simulink model "xpc1_rlti_varx_sqrt"  (Simulink 7.8)
settings: Solver=FixedStepDiscrete  StartTime=0.0  StopTime=150.0  FixedStep=0.005  RelTol=1e-3
libraries: xpclib x3, cstblocks x2, xpcnilib x2, simulink x1
settings Model: Creator=IVO  LastModifiedBy=pietergebraad  SimulationMode=external  BufferReuse=off
settings OptimizationCC: BlockReduction=off  OptimizeBlockIOStorage=off  BufferReuse=off  ExpressionFolding=off  LocalBlockOutputs=off
settings DebuggingCC: FcnCallInpInsideContextMsg=Use local settings  StrictBusMsg=Warning
settings HardwareCC: ProdIntDivRoundTo=Zero  ProdEndianess=LittleEndian  ProdHWDeviceType=Generic->32-bit x86 compatible
settings SFSimCC: SFSimEnableDebug=off  SimParseCustomCode=off
settings RTWCC: SystemTargetFile=xpctarget.tlc  TemplateMakefile=xpc_default_tmf  Description=xPC Target  ProcessScript=xpctarget_make_rtw_hook  RTWCompilerOptimization=On
settings xpcTargetCC: TargetFcnLib=ansi_tfl_table_tmw.mat  TargetFunctionLibrary=XPC_BLAS  CodeExecutionProfiling=off  ParMdlRefBuildCompliant=on  ConcurrentExecutionCompliant=on  CombineSignalStateStructs=off  PortableWordSizes=off  xPCTaskExecutionProfile=off  xPCRL32EventNumber=5000  xPCisDefaultEnv=off  xPCTargetPCEnvName=TargetPC1  xPCLoadParamSetFile=off  xPCConcurrentTasks=off  xPCEnableSFAnimation=off

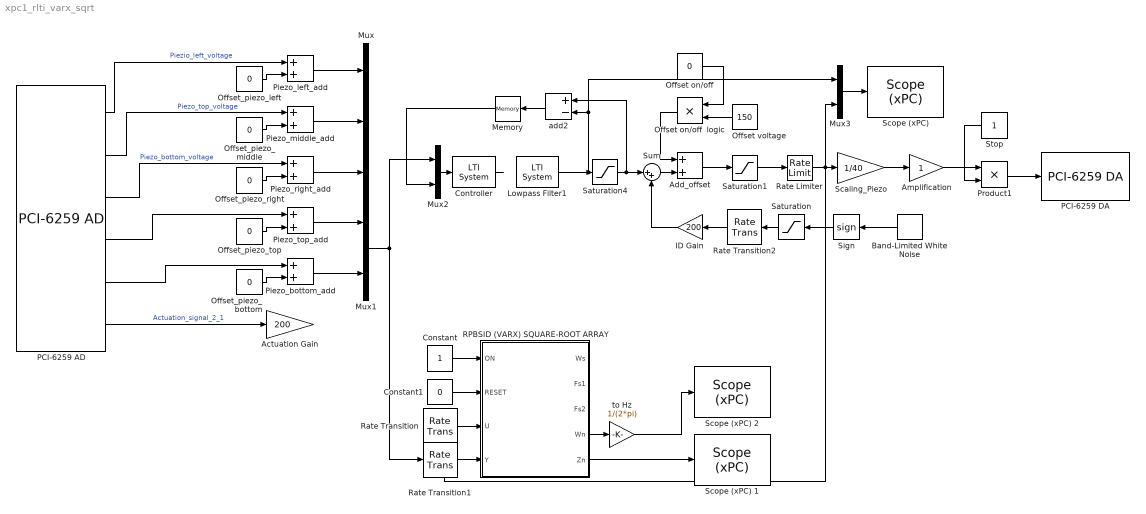
== system xpc1_rlti_varx_sqrt ==
  Actuation Gain : Gain  Gain=200
  Add_offset : Sum
  Amplification : Gain
  Band-Limited White Noise : simulink/Sources/Band-Limited White Noise  Cov=1  Ts=0.25  seed=[23341]
  Constant : Constant
  Constant1 : Constant  Value=0
  Controller : cstblocks/LTI System  sys=Cs  IC=[]
  ID Gain : Gain  Gain=200
  Lowpass Filter1 : cstblocks/LTI System  sys=Fs  IC=[]
  Memory : Memory
  Mux : Mux  Inputs=3
  Mux1 : Mux  Inputs=2
  Mux2 : Mux  Inputs=2
  Mux3 : Mux  Inputs=2
  Offset on/off : Constant  Value=0  OutDataTypeStr=boolean
  Offset on/off  logic : Product  RndMeth=Zero
  Offset voltage : Constant  Value=150
  Offset_piezo_bottom : Constant  Value=0
  Offset_piezo_left : Constant  Value=0
  Offset_piezo_middle : Constant  Value=0
  Offset_piezo_right : Constant  Value=0
  Offset_piezo_top : Constant  Value=0
  PCI-6259 AD : xpcnilib/A//D/M Series/PCI-6259 AD  channel=[17,18,19,20,21,22]  range=[10]  coupling=[0]  scantime=5e-6  sampletime=0.005  slot=-1
  PCI-6259 DA : xpcnilib/D//A/M Series/PCI-6259 DA  channel=[3]  range=[10]  reset=[1]  initValue=[0]  sampletime=0.005  slot=-1
  Piezo_bottom_add : Sum
  Piezo_left_add : Sum
  Piezo_middle_add : Sum
  Piezo_right_add : Sum
  Piezo_top_add : Sum
  Product1 : Product  RndMeth=Zero
  RPBSID (VARX) SQUARE-ROOT ARRAY : MATLAB Function  TreatAsAtomicUnit=on
  Rate Limiter : RateLimiter  RisingSlewLimit=10000  FallingSlewLimit=-10000  SampleTimeMode=inherited
  Rate Transition : RateTransition  Integrity=off  Deterministic=off  OutPortSampleTime=0.05
  Rate Transition1 : RateTransition  Integrity=off  Deterministic=off  OutPortSampleTime=0.05
  Rate Transition2 : RateTransition
  Saturation : Saturate  UpperLimit=1  LowerLimit=-1
  Saturation1 : Saturate  UpperLimit=290  LowerLimit=-290
  Saturation4 : Saturate  UpperLimit=290  LowerLimit=-290
  Scaling_Piezo : Gain  Gain=1/40
  "Scope (xPC) " : xpclib/Misc./Scope (xPC)   scopeno=1  scopetype=Target  autostart=on  viewmode=Graphical rolling  formatstr='%15.6f'  grid=on  ylimits=[-300,300]  nosamples=600  noprepostsamples=0  interleave=1  triggermode=FreeRun  triggersignal=1  triggerlevel=0.0  triggerslope=Either  triggerscope=1  triggersample=0  filename=data.dat  mode=Lazy  writesize=512  autorestart=off  dynamicfilemode=off  maxwritefilesize=512*1024^2
  Scope (xPC) 1 : xpclib/Misc./Scope (xPC)   scopeno=2  scopetype=Target  autostart=on  viewmode=Graphical rolling  formatstr='%15.6f'  grid=on  ylimits=[-0.05,0.03]  nosamples=60  noprepostsamples=0  interleave=1  triggermode=FreeRun  triggersignal=1  triggerlevel=0.0  triggerslope=Either  triggerscope=1  triggersample=0  filename=data.dat  mode=Lazy  writesize=512  autorestart=off  dynamicfilemode=off  maxwritefilesize=512*1024^2
  Scope (xPC) 2 : xpclib/Misc./Scope (xPC)   scopeno=3  scopetype=Target  autostart=on  viewmode=Graphical rolling  formatstr='%15.6f'  grid=on  ylimits=[2,3.5]  nosamples=60  noprepostsamples=0  interleave=1  triggermode=FreeRun  triggersignal=1  triggerlevel=0.0  triggerslope=Either  triggerscope=1  triggersample=0  filename=data.dat  mode=Lazy  writesize=512  autorestart=off  dynamicfilemode=off  maxwritefilesize=512*1024^2
  Sign : Signum
  Stop : Constant
  Sum : Sum  Inputs=|++
  add2 : Sum  Inputs=+-
  to Hz : Gain  Gain=1/(2*pi)
  wires:
  Offset_piezo_left/1 -> Piezo_left_add/2
  PCI-6259 AD/1 -> Piezo_left_add/1  "Piezio_left_voltage"
  Offset_piezo_middle/1 -> Piezo_middle_add/2
  Offset_piezo_right/1 -> Piezo_right_add/2
  PCI-6259 AD/6 -> Actuation Gain/1  "Actuation_signal_2_1"
  Offset_piezo_top/1 -> Piezo_top_add/2
  Offset_piezo_bottom/1 -> Piezo_bottom_add/2
  Piezo_left_add/1 -> Mux/1
  Piezo_middle_add/1 -> Mux/2
  Piezo_right_add/1 -> Mux/3
  Piezo_top_add/1 -> Mux1/1
  Piezo_bottom_add/1 -> Mux1/2
  PCI-6259 AD/2 -> Piezo_middle_add/1  "Piezo_top_voltage"
  PCI-6259 AD/3 -> Piezo_right_add/1  "Piezo_bottom_voltage"
  PCI-6259 AD/4 -> Piezo_top_add/1
  PCI-6259 AD/5 -> Piezo_bottom_add/1
  Scaling_Piezo/1 -> Amplification/1
  Saturation1/1 -> Rate Limiter/1
  Amplification/1 -> Product1/1
  Product1/1 -> PCI-6259 DA/1
  Stop/1 -> Product1/2
  Rate Limiter/1 -> Mux3/2, Scaling_Piezo/1, Rate Transition/1
  Add_offset/1 -> Saturation1/1
  Offset on/off  logic/1 -> Add_offset/1
  Offset on/off/1 -> Offset on/off  logic/1
  Offset voltage/1 -> Offset on/off  logic/2
  Controller/1 -> ?
  Mux1/1 -> Mux2/1, Rate Transition1/1
  Mux3/1 -> "Scope (xPC) "/1
  Lowpass Filter1/1 -> add2/2, Mux3/1, Saturation4/1
  add2/1 -> Memory/1
  Saturation4/1 -> add2/1, Sum/1
  Memory/1 -> Mux2/2
  Constant/1 -> RPBSID (VARX) SQUARE-ROOT ARRAY/1(ON)
  RPBSID (VARX) SQUARE-ROOT ARRAY/4(Wn) -> to Hz/1
  to Hz/1 -> Scope (xPC) 2/1
  Constant1/1 -> RPBSID (VARX) SQUARE-ROOT ARRAY/2(RESET)
  RPBSID (VARX) SQUARE-ROOT ARRAY/5(Zn) -> Scope (xPC) 1/1
  Rate Transition/1 -> RPBSID (VARX) SQUARE-ROOT ARRAY/3(U)
  Rate Transition1/1 -> RPBSID (VARX) SQUARE-ROOT ARRAY/4(Y)
  Band-Limited White Noise/1 -> Sign/1
  Saturation/1 -> Rate Transition2/1
  Sign/1 -> Saturation/1
  Rate Transition2/1 -> ID Gain/1
  Mux2/1 -> Controller/1
  ID Gain/1 -> Sum/2
  Sum/1 -> Add_offset/2

== matlab function RPBSID (VARX) SQUARE-ROOT ARRAY ==
  data: ON input double; RESET input double; Ws output double; Fs1 output double; Fs2 output double; U input double; Y input double size=2; Wn output double; Zn output double; W parameter double
function [Ws,Fs1,Fs2,Wn,Zn] = rpbsid(ON,RESET,U,Y,W)
%RPBSID Closed-loop recursive predictor-based subspace identification (VARX)

% Input definitions
% U input sample
% Y output sample
% W weight matrix (from workspace)
% Du input scaling matrix from sigscale (from workspace)
% Dy output scaling matric from sigscale (from workspace)

% Common paremeters
r = 1;         % number if inpuh
l = 2;         % number of outpuh
m = l+r;
n = 7;         % number of states
Ts = 0.05;      % sample time

% Parameters for identification
p = 50;        % past window
f = 50;        % future window
noD = 0;       % no direct feedtrough
off = 1;       % remove offset in Markov estimation
weight = 0;    % apply transformation filter

% Parameters for adaptive filters
lambda1 = 0.999; % initial forgetting factor (~= 1 - 2/window)
lambda2 = 0.999; % initial forgetting factor (~= 1 - 2/window)
lambda3 = 0.999; % initial forgetting factor (~= 1 - 2/window)
ireg1 = 100;     % initial regularisation
ireg2 = 1e-6;    % initial regularisation
ireg3 = 1e-6;    % initial regularisation
reg1 = 1;        % initial regularisation

% Initialization
startA = 3;

% Initialize if needed
persistent Plk VARX LK Pcd Pabk ABK CD U1 Y1 X X1 Zp w k start saw
if isempty(Plk)
    % Initialisation of Markov estimation problem
    if noD
        if off
            Plk = (1/sqrt(ireg1)).*eye(p*m+1);
            VARX = zeros(l,p*m+1);
        else
            Plk = (1/sqrt(ireg1)).*eye(p*m);
            VARX = zeros(l,p*m);
        end
    else
        if off
            Plk = (1/sqrt(ireg1)).*eye(p*m+r+1);
            VARX = zeros(l,p*m+r+1);
        else
            Plk = (1/sqrt(ireg1)).*eye(p*m+r);
            VARX = zeros(l,p*m+r);
        end
    end
    saw = 0;
    
    % Initialisation of the LambdaKappa
    LK = zeros(f*l,m*p);
    
    % Initialisation the estimate of ABK
    Pabk = (1/sqrt(ireg2)).*eye(n+r+l);
    ABK = [zeros(n) zeros(n,r) zeros(n,l)];
    
    if noD
        % Initialisation the estimate of CD
        Pcd = (1/sqrt(ireg3)).*eye(n);
        CD = zeros(l,n);
    else
        % Initialisation the estimate of CD and e
        Pcd = (1/sqrt(ireg3)).*eye(n+r);
        CD = [zeros(l,n) zeros(l,r)];
    end

    % Store vectors for next iteration
    Y1 = zeros(l,1);
    U1 = zeros(r,1);
    X1 = zeros(n,1);
    X = zeros(n,1);
    Zp = zeros(p*m,1); 
    
    % Frequency grid
    w = logspace(-1,1,300);
    k = 1;
    start = 1;
end

% Start RPBSID iff ON is set
if ON > 0.5
    
    % Scale input and output
    U = U./100;
    Y = Y;
    
    % New signal vector
    Zp(1:(p-1)*m,1) = Zp(m+1:p*m,1);
    Zp((p-1)*m+1:p*m,1) = [U1; Y1];
    if noD
        if off
            Z = [Zp; 1];
        else
            Z = Zp;
        end
    else
        if off
            Z = [Zp; U; 1];
        else
            Z = [Zp; U];
        end
    end

    if (start < 0.5) || (k >= p)
        % Solve Markov estimation problem recursively
        if reg1 ~= 0
            [VARX,Plk,saw] = inverseQRreg(Z,Y,VARX,Plk,lambda1,reg1,saw);
        else
            [VARX,Plk] = inverseQR(Z,Y,VARX,Plk,lambda1);
        end
    end
    
    if (start < 0.5) || (k >= startA*p)
        % Construction of LambdaKappa
        LK = zeros(f*l,p*m);
        if ~weight
            for i = 0:f-1
                for h = 0:p-i-1
                    LK(i*l+(1:l),(i+h)*m+(1:m)) = VARX(:,h*m+(1:m));
                end
            end
        else
            for i = 0:f-1
                for h = 0:p-i-1
                    LK(i*l+(1:l),(i+h)*m+(1:m)) = VARX(:,h*m+(1:m));
                end
                if i ~= 0
                    for j = 0:i-1
                        LK(i*l+(1:l),:) = LK(i*l+(1:l),:) + VARX(:,(p-i+j)*m+r+(1:l))*LK(j*l+(1:l),:);
                    end
                end
            end
        end
        
        % The estimation of the state vector
        X = W*LK*Zp;
    end
    
    if (start < 0.5) || (k >= startA*p+1)
        % The estimation of the system matrices
        if noD
            [CD,Pcd] = inverseQR(X1,Y1,CD,Pcd,lambda2);
            R1 = Y1-CD*X1;
        else
            [CD,Pcd] = inverseQR([X1; U1],Y1,CD,Pcd,lambda2);
            R1 = Y1-CD*[X1; U1];
        end
        [ABK,Pabk] = inverseQR([X1; U1; R1],X,ABK,Pabk,lambda3);
    end
        
    % Store vectors and matrices for next iteration
    if (start < 0.5) || (k >= startA*p)
        X1 = X;
    end
    Y1 = Y;
    U1 = U;
end

% Store state-space matrices
A = ABK(:,1:n);
B = ABK(:,n+1:n+r);
C = CD(:,1:n);
if noD
    D = zeros(l,r);
else
    D = CD(:,n+1:end);
end
K = ABK(:,n+r+1:n+r+l);

% Calculate damping and frequencies
[Wn,Zn] = damp(A,Ts);

% Calculate frequency response
Ws = w(k);
Fs = real(abs(C*((exp(sqrt(complex(-1))*Ts*Ws*2*pi).*eye(n) - A)\B)+D));
Ws = log10(Ws);
if Fs(1) < 1e-5
    Fs1 = -100;
else
    Fs1 = 20*log10(Fs(1));
end
if Fs(2) < 1e-5
    Fs2 = -100;
else
    Fs2 = 20*log10(Fs(2));
end

% Update counter
if k >= length(w)
    start = 0;
    k = 1;
else
    k = k+1;
end

end % END RPBSID


function [theta,P,saw,R] = inverseQRreg(z,y,theta,P,lambda,reg,saw)
%INVERSEQR Square-Root Recursive Least Squares update (inverse QR)
[mz,nz] = size(z);

% Do regularization update first
eta = zeros(mz,nz);
if saw > (mz-0.5)
   saw = 1;
else
   saw = saw + 1; 
end
eta(saw) = sqrt((1-lambda^mz)*reg);
M = [eye(nz) eta'*P; zeros(mz,nz) P];
for i = (size(P,2)+nz):-1:2
    % determine Givens rotation parameters
    if M(1,i) == 0
    elseif M(1,1) == 0
        % swap
        h = M(:,i);
        M(:,i) = -M(:,1);
        M(:,1) = h;
    else
        % determine Givens rotation parameters
        rho = M(1,i)/M(1,1);
        c = sqrt(1+abs(rho)^2);
        
        % apply givens rotation using mixed-downdating (more numeric stable)
        M(:,1) = (M(:,1) + rho.*M(:,i))./c;
        M(:,i) = -rho.*M(:,1) + c.*M(:,i);
    end
end
P = M(nz+1:end,nz+1:end);

% Do data update
zp = z'*P;
M = [eye(nz) (zp)./sqrt(lambda); zeros(mz,nz) P./sqrt(lambda)];
for i = (size(P,2)+nz):-1:2
    % determine Givens rotation parameters
    if M(1,i) == 0
    elseif M(1,1) == 0
        % swap
        h = M(:,i);
        M(:,i) = -M(:,1);
        M(:,1) = h;
    else
        % determine Givens rotation parameters
        rho = M(1,i)/M(1,1);
        c = sqrt(1+abs(rho)^2);
        
        % apply givens rotation using mixed-downdating (more numeric stable)
        M(:,1) = (M(:,1) + rho.*M(:,i))./c;
        M(:,i) = -rho.*M(:,1) + c.*M(:,i);
    end
end
G = M(nz+1:end,1:nz)/M(1:nz,1:nz);
P = M(nz+1:end,nz+1:end);
E = y - theta*z;
theta = theta + E*G';
if nargout == 3
    R = norm(y - theta*z);
end
end

function [theta,P,R] = inverseQR(z,y,theta,P,lambda)
%INVERSEQR Square-Root Recursive Least Squares update (inverse QR)

[mz,nz] = size(z);
zp = z'*P;
M = [eye(nz) (zp)./sqrt(lambda); zeros(mz,nz) P./sqrt(lambda)];
for i = (size(P,2)+nz):-1:2
    % determine Givens rotation parameters
    if M(1,i) == 0
    elseif M(1,1) == 0
        % swap
        h = M(:,i);
        M(:,i) = -M(:,1);
        M(:,1) = h;
    else
        % determine Givens rotation parameters
        rho = M(1,i)/M(1,1);
        c = sqrt(1+abs(rho)^2);
        
        % apply givens rotation using mixed-downdating (more numeric stable)
        M(:,1) = (M(:,1) + rho.*M(:,i))./c;
        M(:,i) = -rho.*M(:,1) + c.*M(:,i);
    end
end
G = M(nz+1:end,1:nz)/M(1:nz,1:nz);
P = M(nz+1:end,nz+1:end);
E = y - theta*z;
theta = theta + E*G';
if nargout == 3
    R = norm(y - theta*z);
end
end


function [wn,z] = damp(a,h)
%DAMP  Natural frequency and damping

% Calculate eigenvalues
r = eig(a);
[~,I] = sort(real(r));
r = r(I);

% Discrete: compute equivalent S-plane poles
if any(r) == 0
    z = zeros(size(r));
    wn = zeros(size(r));
else
    s = log(r)/h;
    f = abs(s);
    wn = f;
    z = -real(s)./f;
end
end

%% UNCOMMENT THE LATTER FOR OLDER MATLAB VERSIONS

% function y = log10(x)
% %LOG10  Common (base 10) logarithm.
% y = log(x)/log(10);
% end

% function E = eig(A)
% % Compute eigenvalues of matrix
% tol = 1e-4;
% maxit = 20;
% n = size(A,1);
% C = complex(A,zeros(n));
% A1 = C(n,n);
% E = complex(zeros(n,1),zeros(n,1));
% I = eye(n);
% for k2 = n:-1:2
%     k = 1;
%     brk = 0;
%     while k <= maxit && brk <= 0.5
%         mu = qrshift(C(k2+(-1:0),k2+(-1:0)));
%         M = (C - mu(1).*I);
%         [Q,R] = qr(M);
%         C = (R*Q + mu(1).*I);
%         if abs(abs(A1)-abs(C(k2,k2))) < tol
%             brk = 1;
%             A1 = C(k2-1,k2-1);
%         else
%             A1 = C(k2,k2);
%         end
%         k = k+1;
%     end
%     E(k2) = C(k2,k2);
%     C(k2,1:n) = 0;
%     C(1:n,k2) = 0;
%     I(k2,k2) = 0;
% end
% E(1) = C(1,1);
% E = sort(E);
% end

% function mu = qrshift(A)
% % Compute the Wilkinson double shift
% 
% trA = A(1,1) + A(2,2);
% detA =  A(1,1)*A(2,2) - A(1,2)*A(2,1);
% 
% mu1 = 0.5*(trA + sqrt(trA^2-4*detA));
% mu2 = 0.5*(trA - sqrt(trA^2-4*detA));
% if abs(abs(A(2,2)) - abs(mu1)) < abs(abs(A(2,2)) - abs(mu2))
%     mu = mu1;
% else
%     mu = mu2;
% end
% end
